simulink model "Kirchhoff_a"  (R2025a)
settings: Solver=VariableStepAuto  StartTime=0.0  StopTime=10.0  RelTol=1e-3
libraries: fl_lib x21, nesl_utility x14
settings Model: Creator=Maria Paz Puerta  LastModifiedBy=Maria Paz Puerta

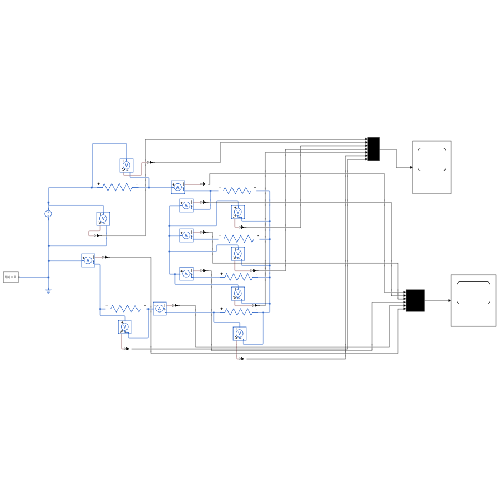
[thumbnail: Simulink's stored preview of the top-level diagram]
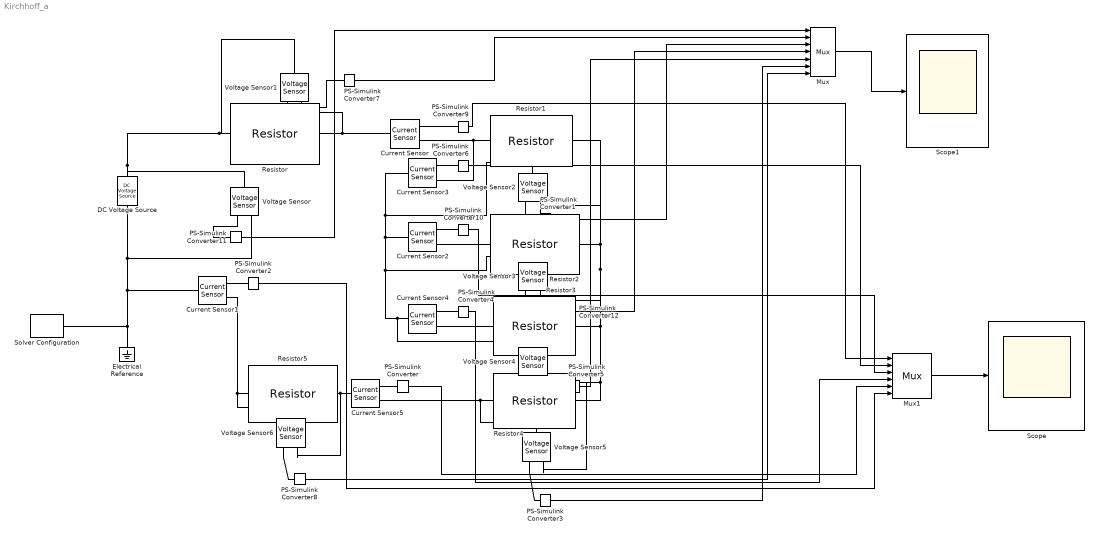
== system Kirchhoff_a ==
  Current Sensor{,1..5} (6 alike) : fl_lib/Electrical/Electrical Sensors/Current Sensor
  DC Voltage Source : fl_lib/Electrical/Electrical Sources/DC Voltage Source  v0=12 V
  Electrical Reference : fl_lib/Electrical/Electrical Elements/Electrical Reference
  Mux : Mux  Inputs=7
  Mux1 : Mux  Inputs=6
  PS-Simulink Converter{,1..12} (13 alike) : nesl_utility/PS-Simulink Converter  PhysicalDomain=network_engine_domain  SubClassName=ps_output  LeftPortType=input  RightPortType=output  PseudoPeriodic=off  Frequencies=[]  VectorFormat=inherit  Unit=inherit  AffineConversion=off
  Resistor : fl_lib/Electrical/Electrical Elements/Resistor  R=82 Ohm  i_specify=off  i_priority=None  i=0 A  i_nominal_specify=off  i_nominal_value=1  i_nominal_unit=A  v_specify=off  v_priority=None  v=0 V  v_nominal_specify=off  v_nominal_value=1  v_nominal_unit=V
  Resistor1 : fl_lib/Electrical/Electrical Elements/Resistor  R=100 Ohm  i_specify=off  i_priority=None  i=0 A  i_nominal_specify=off  i_nominal_value=1  i_nominal_unit=A  v_specify=off  v_priority=None  v=0 V  v_nominal_specify=off  v_nominal_value=1  v_nominal_unit=V
  Resistor2 : fl_lib/Electrical/Electrical Elements/Resistor  R=150 Ohm  i_specify=off  i_priority=None  i=0 A  i_nominal_specify=off  i_nominal_value=1  i_nominal_unit=A  v_specify=off  v_priority=None  v=0 V  v_nominal_specify=off  v_nominal_value=1  v_nominal_unit=V
  Resistor3 : fl_lib/Electrical/Electrical Elements/Resistor  R=330 Ohm  i_specify=off  i_priority=None  i=0 A  i_nominal_specify=off  i_nominal_value=1  i_nominal_unit=A  v_specify=off  v_priority=None  v=0 V  v_nominal_specify=off  v_nominal_value=1  v_nominal_unit=V
  Resistor4 : fl_lib/Electrical/Electrical Elements/Resistor  R=220 Ohm  i_specify=off  i_priority=None  i=0 A  i_nominal_specify=off  i_nominal_value=1  i_nominal_unit=A  v_specify=off  v_priority=None  v=0 V  v_nominal_specify=off  v_nominal_value=1  v_nominal_unit=V
  Resistor5 : fl_lib/Electrical/Electrical Elements/Resistor  R=100 Ohm  i_specify=off  i_priority=None  i=0 A  i_nominal_specify=off  i_nominal_value=1  i_nominal_unit=A  v_specify=off  v_priority=None  v=0 V  v_nominal_specify=off  v_nominal_value=1  v_nominal_unit=V
  Scope : Scope
      settings: ActiveDisplayYMinimum=-0.032491524158539051  ActiveDisplayYMaximum=0.031952383050344021
  Scope1 : Scope
      settings: Title=Voltaje en cada resistencia (Estado estacionario)  ActiveDisplayYMinimum=-7.3436315072270979  ActiveDisplayYMaximum=14.011407305402589  YLabel=Voltaje (V)
  Solver Configuration : nesl_utility/Solver Configuration  PhysicalDomain=network_engine_domain  SubClassName=solver  LeftPortType=input  RightPortType=generic  Tones=[]  Harmonics=[]  SimulateNoise=off  Profile=off  UseLocalSampling=off  EnableSwitchedLinearOptims=on  FrequencyDomain=off  UseCCode=off  RelTol=0.001  AbsTol=0.001  MinStep=1e-09  ToWorkspace=off  RevertToSquareIcSolve=off  NumHomotopyIterations=100  PhasorMode=off  PhasorModeNumHarmonics=1  ConsistencySolver=NEWTON_XTOL_AFTER_FTOL  IndexReductionMethod=DerivativeReplacement  DoDC=off  ResidualTolerance=1e-09  ConsistencyTolSource=GLOBAL  ConsistencyAbsTol=0.001  ConsistencyRelTol=0.001  ConsistencyTolFactor=0.001  UseLocalSolver=off  LocalSolverChoice=NE_BACKWARD_EULER_ADVANCER  ResolveIndetEquations=on  FunctionEvalNumThread=1  LocalSolverSampleTime=0.001  DoFixedCost=off  MaxNonlinIter=3  MaxModeIter=2  ComputeImpulses=off  ImpulseIterations=2  LinearAlgebra=auto  LinearAlgebraNumThread=0  EquationFormulation=NE_TIME_EF  DelaysMemoryBudget=1024  AutomaticFiltering=on  FilteringTimeConstant=0.001  PartitionStorageMethod=AS_NEEDED  PartitionMemoryBudget=1024  PartitionMethod=ROBUST  MultibodyUseLocalSolver=off  MultibodyLocalSolverChoice=ODE1  MultibodyLocalSolverSampleTime=0.001
  Voltage Sensor{,1..6} (7 alike) : fl_lib/Electrical/Electrical Sensors/Voltage Sensor
  wires:
  PS-Simulink Converter11/1 -> Mux/1
  PS-Simulink Converter7/1 -> Mux/2
  Mux/1 -> Scope1/1
  PS-Simulink Converter1/1 -> Mux/3
  PS-Simulink Converter12/1 -> Mux/4
  PS-Simulink Converter5/1 -> Mux/5
  PS-Simulink Converter3/1 -> Mux/6
  PS-Simulink Converter8/1 -> Mux/7
  PS-Simulink Converter9/1 -> Mux1/1
  PS-Simulink Converter6/1 -> Mux1/2
  PS-Simulink Converter10/1 -> Mux1/3
  PS-Simulink Converter4/1 -> Mux1/4
  PS-Simulink Converter/1 -> Mux1/5
  PS-Simulink Converter2/1 -> Mux1/6
  Mux1/1 -> Scope/1
  connections:
  DC Voltage Source/LConn1 -- Voltage Sensor/LConn1 -- Voltage Sensor1/LConn1 -- Resistor/LConn1
  DC Voltage Source/RConn1 -- Electrical Reference/LConn1 -- Solver Configuration/RConn1 -- Current Sensor1/LConn1 -- Voltage Sensor/RConn2
  Resistor1/LConn1 -- Current Sensor/RConn2 -- Current Sensor3/RConn2
  Resistor3/RConn1 -- Voltage Sensor5/RConn2 -- Resistor4/RConn1 -- Voltage Sensor4/RConn2 -- Voltage Sensor3/RConn2 -- Resistor1/RConn1 -- Voltage Sensor2/RConn2 -- Resistor2/RConn1
  Resistor/RConn1 -- Voltage Sensor1/RConn2 -- Current Sensor/LConn1
  Current Sensor2/RConn2 -- Resistor2/LConn1
  Current Sensor4/RConn2 -- Resistor3/LConn1
  Current Sensor2/LConn1 -- Current Sensor3/LConn1 -- Voltage Sensor2/LConn1 -- Voltage Sensor3/LConn1 -- Voltage Sensor4/LConn1 -- Current Sensor4/LConn1
  Resistor5/RConn1 -- Voltage Sensor6/RConn2 -- Current Sensor5/LConn1
  Resistor4/LConn1 -- Voltage Sensor5/LConn1 -- Current Sensor5/RConn2
  Resistor5/LConn1 -- Voltage Sensor6/LConn1 -- Current Sensor1/RConn2
  PS-Simulink Converter10/LConn1 -- Current Sensor2/RConn1
  PS-Simulink Converter9/LConn1 -- Current Sensor/RConn1
  PS-Simulink Converter6/LConn1 -- Current Sensor3/RConn1
  PS-Simulink Converter4/LConn1 -- Current Sensor4/RConn1
  PS-Simulink Converter2/LConn1 -- Current Sensor1/RConn1
  Voltage Sensor2/RConn1 -- PS-Simulink Converter1/LConn1
  Voltage Sensor1/RConn1 -- PS-Simulink Converter7/LConn1
  Voltage Sensor/RConn1 -- PS-Simulink Converter11/LConn1
  PS-Simulink Converter/LConn1 -- Current Sensor5/RConn1
  Voltage Sensor6/RConn1 -- PS-Simulink Converter8/LConn1
  Voltage Sensor5/RConn1 -- PS-Simulink Converter3/LConn1
  Voltage Sensor4/RConn1 -- PS-Simulink Converter5/LConn1
  Voltage Sensor3/RConn1 -- PS-Simulink Converter12/LConn1
